simulink model "Assignment2_group37"  (R2023b)
settings: Solver=FixedStepAuto  StartTime=0.0  StopTime=10.0  FixedStep=1e-3  RelTol=1e-3  EnableMultiTasking=on
undefined symbols (not defined in the file): a, A0, A1, b, c, D0, D1, D10, D11, D12, D13, D2, D3, D4, D5, D6, D7, D8, D9, magnitude, PTA0, PTA1, PTA2, PTB2, PTB23, PTB3, PTB9, PTC16, PTC17, PTC2, PTC3, PTC4, PTD0, PTD1, PTD2, PTD3
libraries: frdmk64flib x19, etargetslib x2, dspstat3 x1, hdlsllib x1
settings Model: ExtModeTrigDuration=5  Creator=aless  LastModifiedBy=aless
settings OptimizationCC: EnhancedBackFolding=on  PassReuseOutputArgsAs=Individual arguments  ZeroExternalMemoryAtStartup=off  ZeroInternalMemoryAtStartup=off  MaxStackSize=64  OptimizeBlockOrder=speed  DifferentSizesBufferReuse=on  OptimizationCustomize=off  EfficientTunableParamExpr=on
settings DebuggingCC: ParameterTunabilityLossMsg=error
settings HardwareCC: ProdBitPerPointer=32  ProdBitPerSizeT=32  ProdBitPerPtrDiffT=32  ProdLargestAtomicInteger=Long  ProdLargestAtomicFloat=Double  ProdWordSize=32  ProdHWDeviceType=ARM Compatible->ARM Cortex
settings SFSimCC: MATLABDynamicMemAlloc=off
settings RTWCC: Description=Embedded Coder  SystemTargetFile=ert.tlc  HardwareBoard=NXP FRDM-K64F  TLCOptions="-aInlineSetEventsForThisBaseRateFcn=TLC_FALSE -aSuppressMultiTaskScheduler=TLC_FALSE  -aRateBasedStepFcn=0"  TemplateMakefile=ert_default_tmf  Toolchain=GNU Tools for ARM Embedded Processors
settings CodeAppCC: ForceParamTrailComments=on  IgnoreCustomStorageClasses=off  OperatorAnnotations=on  SimulinkDataObjDesc=on  SFDataObjDesc=on  InsertBlockDesc=on
settings ERTTargetCC: ExtModeTransport=4  ExtModeMexFile=sendToCommService

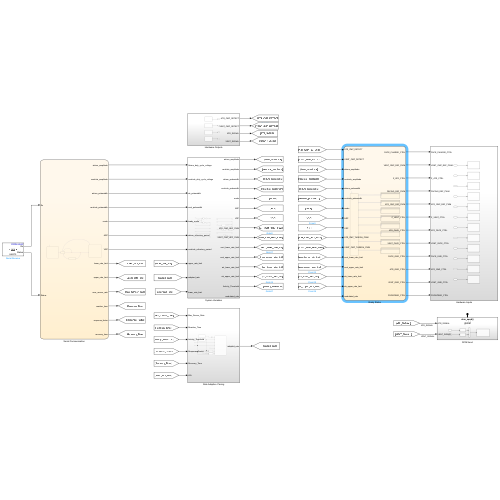
[thumbnail: Simulink's stored preview of the top-level diagram]
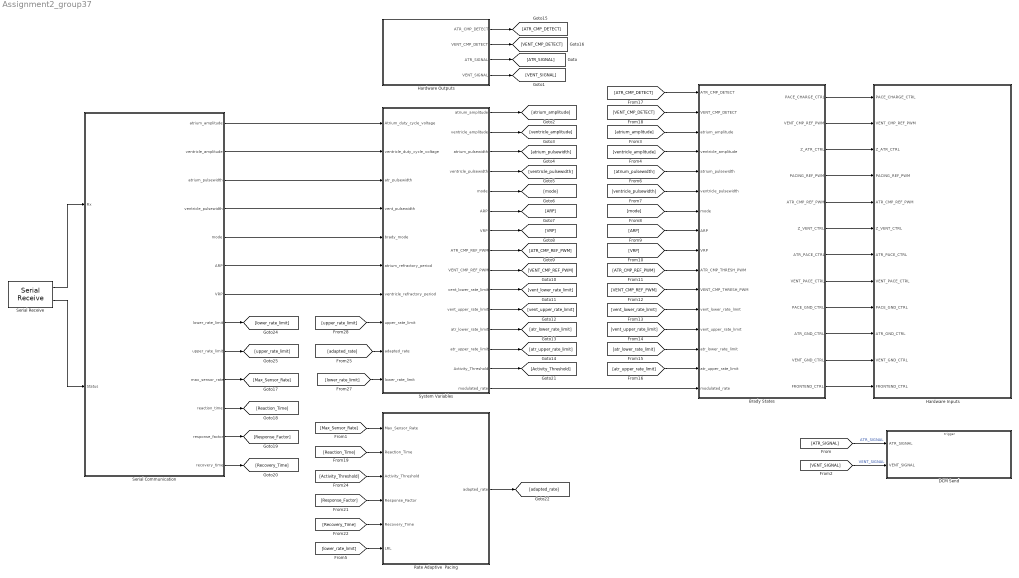
== system Assignment2_group37 ==
  Brady States : Stateflow chart  TreatAsAtomicUnit=on
      settings: PortSchema="{\"entries\":[{\"content\":{\"sides\":[{\"content\":{\"connectorIds\":[\"In1\",\"In2\",\"In3\",\"In4\",\"In5\",\"In6\",\"In7\",\"In8\",\"In9\",\"In10\",\"In11\",\"In12\",\"In13\",\"In14\",\"In15\",\"In16\"]},\"type\":\"ConnectorPlacement.EquallySpacedRectSide\",\"uuid\":\"d1839c8f-6221-46d4-ade1-365648b0880c\"},{\"content\":{\"connectorIds\":[\"Out1\",\"Out2\",\"Out3\",\"Out4\",\"Out5\",\"Out6\",\"Out7\",\"Out8\",\"Out9\",\"Out12\",\"Out10\",\"Out11\"],\"side\":\"RIGHT\"},\"type\":\"ConnectorPlacement.EquallySpacedRectSide\",\"uuid\":\"5469c751-f649-49a4-acaa-2051f4899f66\"},{\"content\":{\"side\":\"TOP\"},\"type\":\"ConnectorPlacement.EquallySpacedRectSide\",\"uuid\":\"ee663bab-8db3-49ac-8698-0304788d9d5e\"},{\"content\":{\"side\":\"BOTTOM\"},\"type\":\"ConnectorPlacement.EquallySpacedRectSide\",\"uuid\":\"7b3ff5b2-4ab8-41cc-b0f7-2e83bde3fafa\"}]},\"type\":\"ConnectorPlacement.EquallySpacedConnector\",\"uuid\":\"0582f962-be2e-4f7f-ab84-ab175671d8de\"}],\"packageUris\":[\"http://schema.mathworks.com/mf0/Connector/R2020b\"],\"version\":\"1.0\"}"
  DCM Send : Subsystem
  Hardware Inputs : Subsystem
  Hardware Outputs : Subsystem
  Rate Adaptive  Pacing : Subsystem
  Serial Communication : Stateflow chart  TreatAsAtomicUnit=on
  Serial Receive : frdmk64flib/Serial Receive  SCIModule=0  Baudrate=uint32(9600)  Parity=None  StopBits=1  HardwareFlowControl=None  ByteOrder=LittleEndian  DataType=uint8  DataLength=48  BlockingMode=off  OutputStatus=on  SampleTime=-1
  System Variables : Subsystem
  wires:
  Brady States/9(PACE_GND_CTRL) -> Hardware Inputs/9(PACE_GND_CTRL)
  Brady States/3(Z_ATR_CTRL) -> Hardware Inputs/3(Z_ATR_CTRL)
  Hardware Outputs/4(VENT_SIGNAL) -> [VENT_SIGNAL]
  Hardware Outputs/3(ATR_SIGNAL) -> [ATR_SIGNAL]
  [Recovery_Time] -> Rate Adaptive  Pacing/5(Recovery_Time)
  [adapted_rate] -> System Variables/9(adapted_rate)
  Serial Receive/1 -> Serial Communication/1(Rx)
  Serial Communication/2(ventricle_amplitude) -> System Variables/2(ventricle_duty_cycle_voltage)
  Serial Communication/7(VRP) -> System Variables/7(ventricle_refractory_period)
  System Variables/8(ATR_CMP_REF_PWM) -> [ATR_CMP_REF_PWM]
  System Variables/7(VRP) -> [VRP]
  System Variables/4(ventricle_pulsewidth) -> [ventricle_pulsewidth]
  System Variables/1(atrium_amplitude) -> [atrium_amplitude]
  [mode] -> Brady States/7(mode)
  System Variables/15(modulated_rate) -> Brady States/16(modulated_rate)
  System Variables/13(atr_upper_rate_limit) -> [atr_upper_rate_limit]
  System Variables/12(atr_lower_rate_limit) -> [atr_lower_rate_limit]
  Brady States/11(FRONTEND_CTRL) -> Hardware Inputs/12(FRONTEND_CTRL)
  Brady States/12(ATR_GND_CTRL) -> Hardware Inputs/10(ATR_GND_CTRL)
  Brady States/8(VENT_PACE_CTRL) -> Hardware Inputs/8(VENT_PACE_CTRL)
  Brady States/7(ATR_PACE_CTRL) -> Hardware Inputs/7(ATR_PACE_CTRL)
  Brady States/2(VENT_CMP_REF_PWM) -> Hardware Inputs/2(VENT_CMP_REF_PWM)
  [ventricle_pulsewidth] -> Brady States/6(ventricle_pulsewidth)
  [ventricle_amplitude] -> Brady States/4(ventricle_amplitude)
  [atr_upper_rate_limit] -> Brady States/15(atr_upper_rate_limit)
  [atr_lower_rate_limit] -> Brady States/14(atr_lower_rate_limit)
  Brady States/10(VENT_GND_CTRL) -> Hardware Inputs/11(VENT_GND_CTRL)
  System Variables/3(atrium_pulsewidth) -> [atrium_pulsewidth]
  System Variables/2(ventricle_amplitude) -> [ventricle_amplitude]
  [Reaction_Time] -> Rate Adaptive  Pacing/2(Reaction_Time)
  [upper_rate_limit] -> System Variables/8(upper_rate_limit)
  [ARP] -> Brady States/8(ARP)
  Hardware Outputs/1(ATR_CMP_DETECT) -> [ATR_CMP_DETECT]
  System Variables/9(VENT_CMP_REF_PWM) -> [VENT_CMP_REF_PWM]
  [Activity_Threshold] -> Rate Adaptive  Pacing/3(Activity_Threshold)
  Brady States/6(Z_VENT_CTRL) -> Hardware Inputs/6(Z_VENT_CTRL)
  Brady States/4(PACING_REF_PWM) -> Hardware Inputs/4(PACING_REF_PWM)
  Serial Communication/13(recovery_time) -> [Recovery_Time]
  System Variables/5(mode) -> [mode]
  [ATR_CMP_DETECT] -> Brady States/1(ATR_CMP_DETECT)
  Serial Communication/10(max_sensor_rate) -> [Max_Sensor_Rate]
  [atrium_pulsewidth] -> Brady States/5(atrium_pulsewidth)
  Serial Communication/3(atrium_pulsewidth) -> System Variables/3(atr_pulsewidth)
  [Max_Sensor_Rate] -> Rate Adaptive  Pacing/1(Max_Sensor_Rate)
  [VENT_CMP_DETECT] -> Brady States/2(VENT_CMP_DETECT)
  System Variables/6(ARP) -> [ARP]
  Brady States/5(ATR_CMP_REF_PWM) -> Hardware Inputs/5(ATR_CMP_REF_PWM)
  System Variables/11(vent_upper_rate_limit) -> [vent_upper_rate_limit]
  [VENT_CMP_REF_PWM] -> Brady States/11(VENT_CMP_THRESH_PWM)
  [lower_rate_limit] -> System Variables/10(lower_rate_limit)
  Serial Receive/2 -> Serial Communication/2(Status)
  Serial Communication/4(ventricle_pulsewidth) -> System Variables/4(vent_pulsewidth)
  System Variables/10(vent_lower_rate_limit) -> [vent_lower_rate_limit]
  [Response_Factor] -> Rate Adaptive  Pacing/4(Response_Factor)
  Rate Adaptive  Pacing/1(adapted_rate) -> [adapted_rate]
  Hardware Outputs/2(VENT_CMP_DETECT) -> [VENT_CMP_DETECT]
  [VRP] -> Brady States/9(VRP)
  Serial Communication/1(atrium_amplitude) -> System Variables/1(Atrium_duty_cycle_voltage)
  [lower_rate_limit] -> Rate Adaptive  Pacing/6(LRL)
  Serial Communication/12(response_factor) -> [Response_Factor]
  Serial Communication/11(reaction_time) -> [Reaction_Time]
  Serial Communication/8(lower_rate_limit) -> [lower_rate_limit]
  Serial Communication/5(mode) -> System Variables/5(brady_mode)
  [ATR_SIGNAL] -> DCM Send/1(ATR_SIGNAL)  "ATR_SIGNAL"
  Brady States/1(PACE_CHARGE_CTRL) -> Hardware Inputs/1(PACE_CHARGE_CTRL)
  [VENT_SIGNAL] -> DCM Send/2(VENT_SIGNAL)  "VENT_SIGNAL"
  [vent_upper_rate_limit] -> Brady States/13(vent_upper_rate_limit)
  [vent_lower_rate_limit] -> Brady States/12(vent_lower_rate_limit)
  [ATR_CMP_REF_PWM] -> Brady States/10(ATR_CMP_THRESH_PWM)
  [atrium_amplitude] -> Brady States/3(atrium_amplitude)
  System Variables/14(Activity_Threshold) -> [Activity_Threshold]
  Serial Communication/6(ARP) -> System Variables/6(atrium_refractory_period)
  Serial Communication/9(upper_rate_limit) -> [upper_rate_limit]

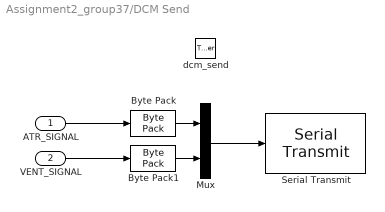
== system Assignment2_group37/DCM Send ==
  ATR_SIGNAL : Inport
  VENT_SIGNAL : Inport  Port=2
  dcm_send : TriggerPort  TriggerType=function-call  IsSimulinkFunction=on  FunctionName=dcm_send  VariantControl=Variant
  Byte Pack : etargetslib/Byte Pack  datatypes={'double'}  byteAlign=1
  Byte Pack1 : etargetslib/Byte Pack  datatypes={'double'}  byteAlign=1
  Mux : Mux  Inputs=2
  Serial Transmit : frdmk64flib/Serial Transmit  SCIModule=0  Baudrate=uint32(9600)  Parity=None  StopBits=1  HardwareFlowControl=None  ByteOrder=LittleEndian  BlockingMode=on  OutputStatus=on
  wires:
  Byte Pack/1 -> Mux/1
  Byte Pack1/1 -> Mux/2
  Mux/1 -> Serial Transmit/1
  ATR_SIGNAL/1 -> Byte Pack/1
  VENT_SIGNAL/1 -> Byte Pack1/1

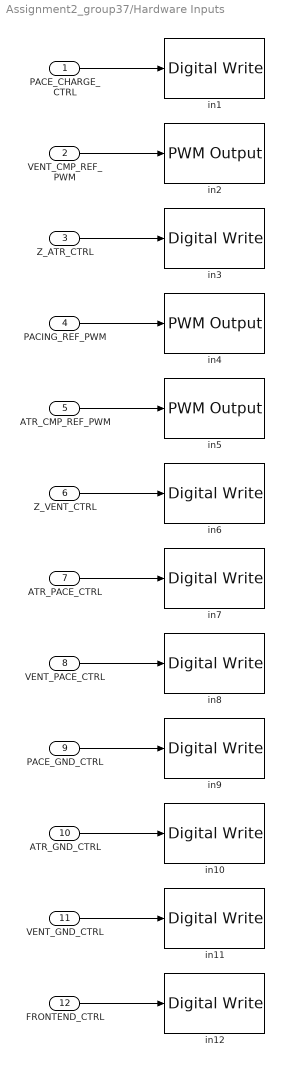
== system Assignment2_group37/Hardware Inputs ==
  PACE_CHARGE_CTRL : Inport
  VENT_CMP_REF_PWM : Inport  Port=2
  Z_ATR_CTRL : Inport  Port=3
  PACING_REF_PWM : Inport  Port=4
  ATR_CMP_REF_PWM : Inport  Port=5
  Z_VENT_CTRL : Inport  Port=6
  ATR_PACE_CTRL : Inport  Port=7
  VENT_PACE_CTRL : Inport  Port=8
  PACE_GND_CTRL : Inport  Port=9
  ATR_GND_CTRL : Inport  Port=10
  VENT_GND_CTRL : Inport  Port=11
  FRONTEND_CTRL : Inport  Port=12
  in1 : frdmk64flib/Digital Write  Whichpin=PTB9 (D2)
  in10 : frdmk64flib/Digital Write  Whichpin=PTD2 (D11)
  in11 : frdmk64flib/Digital Write  Whichpin=PTD3 (D12)
  in12 : frdmk64flib/Digital Write  Whichpin=PTD1 (D13)
  in2 : frdmk64flib/PWM Output  Whichpin=PTA1 (D3)  InitialFrequency=2000  InitialDutyCycle=30
  in3 : frdmk64flib/Digital Write  Whichpin=PTB23 (D4)
  in4 : frdmk64flib/PWM Output  Whichpin=PTA2 (D5)  InitialFrequency=2000  InitialDutyCycle=30
  in5 : frdmk64flib/PWM Output  Whichpin=PTC2 (D6)  InitialFrequency=2000  InitialDutyCycle=30
  in6 : frdmk64flib/Digital Write  Whichpin=PTC3 (D7)
  in7 : frdmk64flib/Digital Write  Whichpin=PTA0 (D8)
  in8 : frdmk64flib/Digital Write  Whichpin=PTC4 (D9)
  in9 : frdmk64flib/Digital Write  Whichpin=PTD0 (D10)
  wires:
  ATR_GND_CTRL/1 -> in10/1
  PACING_REF_PWM/1 -> in4/1
  Z_VENT_CTRL/1 -> in6/1
  VENT_GND_CTRL/1 -> in11/1
  VENT_PACE_CTRL/1 -> in8/1
  ATR_CMP_REF_PWM/1 -> in5/1
  FRONTEND_CTRL/1 -> in12/1
  PACE_CHARGE_CTRL/1 -> in1/1
  ATR_PACE_CTRL/1 -> in7/1
  PACE_GND_CTRL/1 -> in9/1
  Z_ATR_CTRL/1 -> in3/1
  VENT_CMP_REF_PWM/1 -> in2/1

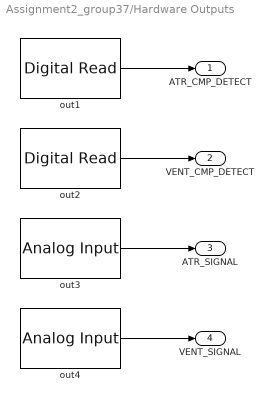
== system Assignment2_group37/Hardware Outputs ==
  out1 : frdmk64flib/Digital Read  Whichpin=PTC16 (D0)  SampleTime=-1
  out2 : frdmk64flib/Digital Read  Whichpin=PTC17 (D1)  SampleTime=-1
  out3 : frdmk64flib/Analog Input  Whichpin=PTB2 (A0)  SampleTime=-1
  out4 : frdmk64flib/Analog Input  Whichpin=PTB3 (A1)  SampleTime=-1
  ATR_CMP_DETECT : Outport
  VENT_CMP_DETECT : Outport  Port=2
  ATR_SIGNAL : Outport  Port=3
  VENT_SIGNAL : Outport  Port=4
  wires:
  out1/1 -> ATR_CMP_DETECT/1
  out2/1 -> VENT_CMP_DETECT/1
  out3/1 -> ATR_SIGNAL/1
  out4/1 -> VENT_SIGNAL/1

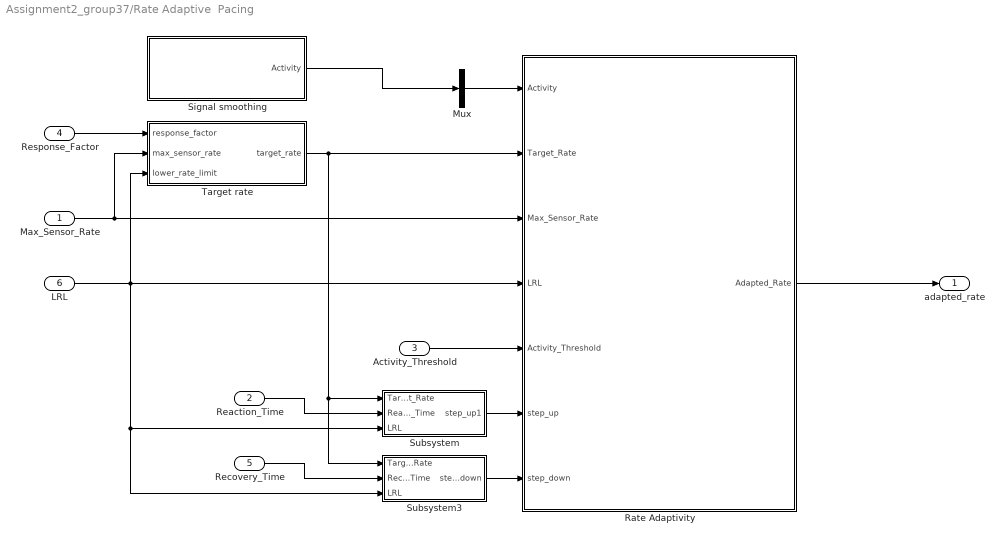
== system Assignment2_group37/Rate Adaptive  Pacing ==
  Max_Sensor_Rate : Inport
  Reaction_Time : Inport  Port=2
  Activity_Threshold : Inport  Port=3
  Response_Factor : Inport  Port=4
  Recovery_Time : Inport  Port=5
  LRL : Inport  Port=6
  Mux : Mux  Inputs=1
  Rate Adaptivity : Stateflow chart  TreatAsAtomicUnit=on
  Signal smoothing : Subsystem
  Subsystem : Subsystem
  Subsystem3 : Subsystem
  Target rate : Subsystem
  adapted_rate : Outport
  wires:
  Activity_Threshold/1 -> Rate Adaptivity/5(Activity_Threshold)
  Mux/1 -> Rate Adaptivity/1(Activity)
  Response_Factor/1 -> Target rate/1(response_factor)
  Signal smoothing/1(Activity) -> Mux/1
  Reaction_Time/1 -> Subsystem/2(Reaction_Time)
  Max_Sensor_Rate/1 -> Target rate/2(max_sensor_rate), Rate Adaptivity/3(Max_Sensor_Rate)
  LRL/1 -> Rate Adaptivity/4(LRL), Subsystem/3(LRL), Subsystem3/3(LRL), Target rate/3(lower_rate_limit)
  Subsystem/1(step_up1) -> Rate Adaptivity/6(step_up)
  Recovery_Time/1 -> Subsystem3/2(Recovery_Time)
  Subsystem3/1(step_down) -> Rate Adaptivity/7(step_down)
  Rate Adaptivity/1(Adapted_Rate) -> adapted_rate/1
  Target rate/1(target_rate) -> Rate Adaptivity/2(Target_Rate), Subsystem3/1(Target_Rate), Subsystem/1(Target_Rate)

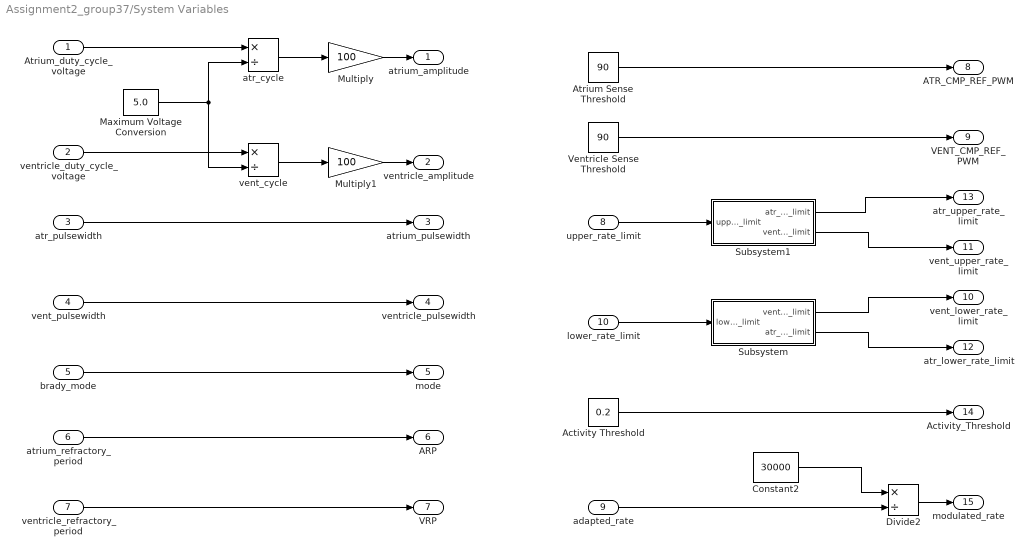
== system Assignment2_group37/System Variables ==
  Atrium_duty_cycle_voltage : Inport
  ventricle_duty_cycle_voltage : Inport  Port=2
  atr_pulsewidth : Inport  Port=3
  vent_pulsewidth : Inport  Port=4
  brady_mode : Inport  Port=5  PortDimensions=8
  atrium_refractory_period : Inport  Port=6
  ventricle_refractory_period : Inport  Port=7
  upper_rate_limit : Inport  Port=8
  adapted_rate : Inport  Port=9
  lower_rate_limit : Inport  Port=10  OutDataTypeStr=double
  Activity Threshold : Constant  Value=0.2  OutDataTypeStr=double
  Atrium Sense Threshold : Constant  Value=90
  Constant2 : Constant  Value=30000
  Divide2 : Product  Inputs=*/
  Maximum Voltage Conversion : Constant  Value=5.0
  Multiply : Gain  Gain=100
  Multiply1 : Gain  Gain=100
  Subsystem : Subsystem
  Subsystem1 : Subsystem
  Ventricle Sense Threshold : Constant  Value=90
  atr_cycle : Product  Inputs=*/
  vent_cycle : Product  Inputs=*/
  atrium_amplitude : Outport
  ventricle_amplitude : Outport  Port=2
  atrium_pulsewidth : Outport  Port=3  OutDataTypeStr=double
  ventricle_pulsewidth : Outport  Port=4  OutDataTypeStr=double
  mode : Outport  Port=5  PortDimensions=8
  ARP : Outport  Port=6  OutDataTypeStr=double
  VRP : Outport  Port=7  OutDataTypeStr=double
  ATR_CMP_REF_PWM : Outport  Port=8
  VENT_CMP_REF_PWM : Outport  Port=9
  vent_lower_rate_limit : Outport  Port=10
  vent_upper_rate_limit : Outport  Port=11
  atr_lower_rate_limit : Outport  Port=12
  atr_upper_rate_limit : Outport  Port=13
  Activity_Threshold : Outport  Port=14
  modulated_rate : Outport  Port=15
  wires:
  atr_cycle/1 -> Multiply/1
  vent_cycle/1 -> Multiply1/1
  Maximum Voltage Conversion/1 -> vent_cycle/2, atr_cycle/2
  brady_mode/1 -> mode/1
  Atrium_duty_cycle_voltage/1 -> atr_cycle/1
  ventricle_duty_cycle_voltage/1 -> vent_cycle/1
  Atrium Sense Threshold/1 -> ATR_CMP_REF_PWM/1
  Ventricle Sense Threshold/1 -> VENT_CMP_REF_PWM/1
  Activity Threshold/1 -> Activity_Threshold/1
  Multiply1/1 -> ventricle_amplitude/1
  Multiply/1 -> atrium_amplitude/1
  lower_rate_limit/1 -> Subsystem/1(lower_rate_limit)
  Subsystem/1(vent_lower_rate_limit) -> vent_lower_rate_limit/1
  ventricle_refractory_period/1 -> VRP/1
  atrium_refractory_period/1 -> ARP/1
  atr_pulsewidth/1 -> atrium_pulsewidth/1
  vent_pulsewidth/1 -> ventricle_pulsewidth/1
  Subsystem/2(atr_lower_rate_limit) -> atr_lower_rate_limit/1
  adapted_rate/1 -> Divide2/2
  Constant2/1 -> Divide2/1
  Divide2/1 -> modulated_rate/1
  upper_rate_limit/1 -> Subsystem1/1(upper_rate_limit)
  Subsystem1/1(atr_upper_rate_limit) -> atr_upper_rate_limit/1
  Subsystem1/2(vent_upper_rate_limit) -> vent_upper_rate_limit/1

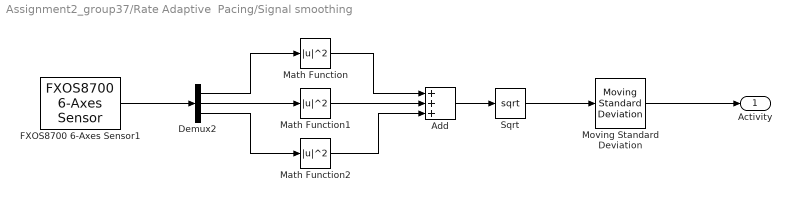
== system Assignment2_group37/Rate Adaptive  Pacing/Signal smoothing ==
  Add : Sum  Inputs=+++
  Demux2 : Demux  Outputs=3
  FXOS8700 6-Axes Sensor1 : frdmk64flib/FXOS8700 6-Axes Sensor  Activesensor=Accelerometer only  ODR=100Hz  HybridODR=400Hz  Accelfullrange=-4g to +4g  SampleTime=1/100
  Math Function : Math  Operator=magnitude^2  SignedPower=on  OutDataTypeStr=double
  Math Function1 : Math  Operator=magnitude^2  SignedPower=on  OutDataTypeStr=double
  Math Function2 : Math  Operator=magnitude^2  SignedPower=on  OutDataTypeStr=double
  Moving Standard Deviation : dspstat3/Moving Standard Deviation  Method=Sliding window  ForgettingFactorPort=off  SpecifyWindowLength=on  WindowLength=128  OverlapLength=127  AllowArbitraryInputLength=off  ForgettingFactor=0.9  SimulateUsing=Code generation
  Sqrt : Sqrt
  Activity : Outport  SourceOfInitialOutputValue=Input signal
  wires:
  Sqrt/1 -> Moving Standard Deviation/1
  FXOS8700 6-Axes Sensor1/1 -> Demux2/1
  Math Function/1 -> Add/1
  Add/1 -> Sqrt/1
  Math Function2/1 -> Add/3
  Demux2/2 -> Math Function1/1
  Math Function1/1 -> Add/2
  Demux2/1 -> Math Function/1
  Demux2/3 -> Math Function2/1
  Moving Standard Deviation/1 -> Activity/1

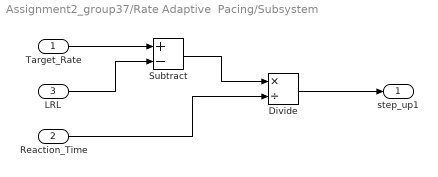
== system Assignment2_group37/Rate Adaptive  Pacing/Subsystem ==
  Target_Rate : Inport
  Reaction_Time : Inport  Port=2
  LRL : Inport  Port=3
  Divide : Product  Inputs=*/
  Subtract : Sum  Inputs=+-
  step_up1 : Outport
  wires:
  Subtract/1 -> Divide/1
  Divide/1 -> step_up1/1
  Target_Rate/1 -> Subtract/1
  LRL/1 -> Subtract/2
  Reaction_Time/1 -> Divide/2

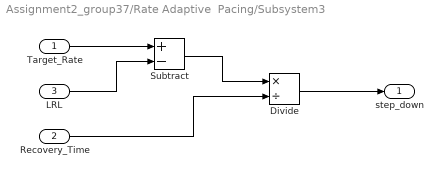
== system Assignment2_group37/Rate Adaptive  Pacing/Subsystem3 ==
  Target_Rate : Inport
  Recovery_Time : Inport  Port=2
  LRL : Inport  Port=3
  Divide : Product  Inputs=*/
  Subtract : Sum  Inputs=+-
  step_down : Outport
  wires:
  Subtract/1 -> Divide/1
  Divide/1 -> step_down/1
  Target_Rate/1 -> Subtract/1
  LRL/1 -> Subtract/2
  Recovery_Time/1 -> Divide/2

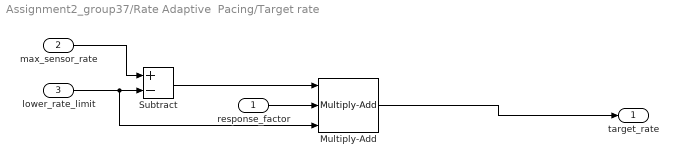
== system Assignment2_group37/Rate Adaptive  Pacing/Target rate ==
  response_factor : Inport
  max_sensor_rate : Inport  Port=2
  lower_rate_limit : Inport  Port=3
  Multiply-Add : hdlsllib/HDL Operations/Multiply-Add  Function=c+(a.*b)  datatype=uint16  RndMeth=Nearest  DoSatur=off  FMA=off
  Subtract : Sum  Inputs=+-
  target_rate : Outport  OutDataTypeStr=uint16  SourceOfInitialOutputValue=Input signal
  wires:
  max_sensor_rate/1 -> Subtract/1
  lower_rate_limit/1 -> Multiply-Add/3, Subtract/2
  Subtract/1 -> Multiply-Add/1
  response_factor/1 -> Multiply-Add/2
  Multiply-Add/1 -> target_rate/1

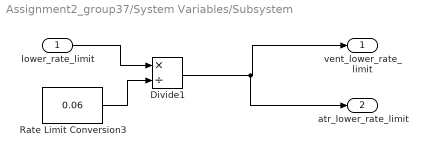
== system Assignment2_group37/System Variables/Subsystem ==
  lower_rate_limit : Inport
  Divide1 : Product  Inputs=*/
  Rate Limit Conversion3 : Constant  Value=0.06
  vent_lower_rate_limit : Outport
  atr_lower_rate_limit : Outport  Port=2
  wires:
  Divide1/1 -> atr_lower_rate_limit/1, vent_lower_rate_limit/1
  lower_rate_limit/1 -> Divide1/1
  Rate Limit Conversion3/1 -> Divide1/2

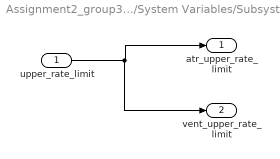
== system Assignment2_group37/System Variables/Subsystem1 ==
  upper_rate_limit : Inport
  atr_upper_rate_limit : Outport
  vent_upper_rate_limit : Outport  Port=2
  wires:
  upper_rate_limit/1 -> vent_upper_rate_limit/1, atr_upper_rate_limit/1

== stateflow chart Assignment2_group37/Serial Communication ==
  state SET_PARAM
    entry:
    mode = typecast(Rx(3:4), 'uint16');
    lower_rate_limit = typecast(Rx(5:6), 'uint16');
    upper_rate_limit = typecast(Rx(7:8), 'uint16');
    ventricle_amplitude = typecast(Rx(9:16), 'double');
    ventricle_pulsewidth = typecast(Rx(17:18), 'uint16');
    VRP = typecast(Rx(19:20), 'uint16');
    atrium_amplitude = typecast(Rx(21:28), 'double');
    atrium_pulsewidth = typecast(Rx(29:30), 'uint16');
    ARP = typecast(Rx(39:40), 'uint16');
    max_sensor_rate = typecast(Rx(41:42), 'uint16');
    reaction_time = typecast(Rx(43:44), 'uint16');
    response_factor = typecast(Rx(45:46), 'uint16');;
    recovery_time = typecast(Rx(47:48), 'uint16');
    update = 1;
  state Initial
    entry:
    mode = 0;
    lower_rate_limit = 60;
    upper_rate_limit = 120;
    reaction_time = 10;
    response_factor = 16;
    recovery_time = 20;
    max_sensor_rate = 180;
    atrium_amplitude = 3.5;
    atrium_pulsewidth = 10;
    ARP = 200;
    ventricle_amplitude = 3.5;
    ventricle_pulsewidth = 10;
    VRP = 200;
  state STANDBY
  state TRANSITION
    entry:
    dcm_send();
  SET_PARAM -> STANDBY
  (default) -> Initial
  (junction 82) -> STANDBY [order 2]
  Initial -> STANDBY
  STANDBY -> (junction 82) : [Status == 0]
  (junction 82) -> (junction 68) [order 1] : [Rx(1) == hex2dec('16')]
  (junction 68) -> SET_PARAM [order 2] : [Rx(2) == hex2dec('55')]
  (junction 68) -> TRANSITION [order 1] : [Rx(2) == hex2dec('22')]
  TRANSITION -> STANDBY
  data: Rx input uint8; Status input uint8; atrium_amplitude output single size=8; ventricle_amplitude output single; atrium_pulsewidth output single; ventricle_pulsewidth output single; mode output uint16; ARP output uint16; VRP output uint16; lower_rate_limit output uint16; upper_rate_limit output uint16; max_sensor_rate output uint16; reaction_time output uint16; response_factor output uint16; recovery_time output uint16

== stateflow chart Assignment2_group37/Brady States ==
  state AOO [group]
    state Charging
      entry:
      %Charge C22
      ATR_PACE_CTRL = false
      VENT_PACE_CTRL = false
      PACING_REF_PWM = atrium_amplitude
      PACE_CHARGE_CTRL = true
      %Discharge C21
      PACE_GND_CTRL = true
      VENT_PACE_CTRL = false
      Z_ATR_CTRL = false
      Z_VENT_CTRL = false
      ATR_PACE_CTRL = false
      ATR_GND_CTRL = true
      VENT_GND_CTRL = false
    state Discharging
      entry:
      %Discharge C22 to charge C21
      PACE_CHARGE_CTRL = false
      PACE_GND_CTRL = true
      VENT_PACE_CTRL = false
      VENT_GND_CTRL = false
      Z_VENT_CTRL = false
      Z_ATR_CTRL = false
      ATR_GND_CTRL = false
      ATR_PACE_CTRL = true
    AOO.Charging -> AOO.Discharging [order 1] : after((60000/atrium_lower_rate_limit)- atrium_pulsewidth,msec)
    AOO.Discharging -> AOO.Charging : after((atrium_pulsewidth),msec)
  state Mode
  state VOO [group]
    state Discharging
      entry:
      %discharge C22 to charge C21
      PACE_CHARGE_CTRL = false
      PACE_GND_CTRL = true
      ATR_PACE_CTRL = false
      ATR_GND_CTRL = false
      Z_VENT_CTRL = false
      Z_ATR_CTRL = false
      VENT_GND_CTRL = false
      VENT_PACE_CTRL = true
    state Charging
      entry:
      %charge C22
      ATR_PACE_CTRL = false
      VENT_PACE_CTRL = false
      PACING_REF_PWM = ventricle_amplitude
      PACE_CHARGE_CTRL = true
      %discharge C21 into ventricle ground
      PACE_GND_CTRL = true
      VENT_PACE_CTRL = false
      Z_ATR_CTRL = false
      Z_VENT_CTRL = false
      ATR_PACE_CTRL = false
      ATR_GND_CTRL = false
      VENT_GND_CTRL = true
    note: after((ventricle_pulsewidth),msec)
    VOO.Discharging -> VOO.Charging
    VOO.Charging -> VOO.Discharging [order 1] : after((60000/ventricle_lower_rate_limit)-ventricle_pulsewidth,msec)
  state AAI [group]
    state Charging
      entry:
      %Turn on sensing
      FRONTEND_CTRL = true
      ATR_CMP_REF_PWM = ATR_CMP_THRESH_PWM
      %Charging capacitor C22
      ATR_PACE_CTRL = false
      VENT_PACE_CTRL = false
      PACING_REF_PWM = atrium_amplitude
      PACE_CHARGE_CTRL = true
      %Discharge C21 into Atrium ground
      PACE_GND_CTRL = true
      VENT_PACE_CTRL = false
      Z_ATR_CTRL = false
      Z_VENT_CTRL = false
      ATR_PACE_CTRL = false
      ATR_GND_CTRL = true
      VENT_GND_CTRL = false
    state Discharging
      entry:
      %discharge C22 to charge C21
      PACE_CHARGE_CTRL = false
      PACE_GND_CTRL = true
      VENT_PACE_CTRL = false
      VENT_GND_CTRL = false
      Z_VENT_CTRL = false
      Z_ATR_CTRL = false
      ATR_GND_CTRL = false
      ATR_PACE_CTRL = true
    state Transition
      %Check for sense outside atrium refractory period
    AAI.Discharging -> AAI.Charging : after(atrium_pulsewidth, msec)
    AAI.Charging -> AAI.Transition [order 1] : after(ARP, msec)
    AAI.Transition -> AAI.Discharging [order 2] : after((60000/atrium_lower_rate_limit) - atrium_pulsewidth - ARP,msec)
    AAI.Transition -> AAI.Charging [order 1] : [ATR_CMP_DETECT == true]
  state VVI [group]
    state Charging
      entry:
      %Turn sensing on
      FRONTEND_CTRL = true
      VENT_CMP_REF_PWM = VENT_CMP_THRESH_PWM
      %Charging C22
      ATR_PACE_CTRL = false
      VENT_PACE_CTRL = false
      PACING_REF_PWM = ventricle_amplitude
      PACE_CHARGE_CTRL = true
      %Charge release of capacitor C21 into Ventricle ground
      PACE_GND_CTRL = true
      VENT_PACE_CTRL = false
      Z_ATR_CTRL = false
      Z_VENT_CTRL = false
      ATR_PACE_CTRL = false
      ATR_GND_CTRL = false
      VENT_GND_CTRL = true
    state Discharging
      entry:
      %discharge C22 to charge C21
      PACE_CHARGE_CTRL = false
      PACE_GND_CTRL = true
      ATR_PACE_CTRL = false
      ATR_GND_CTRL = false
      Z_VENT_CTRL = false
      Z_ATR_CTRL = false
      VENT_GND_CTRL = false
      VENT_PACE_CTRL = true
    state Transition
      %Check for sense outside atrium refractory period
    VVI.Discharging -> VVI.Charging : after(ventricle_pulsewidth, msec)
    VVI.Charging -> VVI.Transition [order 1] : after(VRP, msec)
    VVI.Transition -> VVI.Discharging [order 2] : after((60000/ventricle_lower_rate_limit) - ventricle_pulsewidth - VRP,msec)
    VVI.Transition -> VVI.Charging [order 1] : [VENT_CMP_DETECT == true]
  state AOOR [group]
    state Charging
      entry:
      %Charge C22
      ATR_PACE_CTRL = false
      VENT_PACE_CTRL = false
      PACING_REF_PWM = atrium_amplitude
      PACE_CHARGE_CTRL = true
      %Discharge C21
      PACE_GND_CTRL = true
      VENT_PACE_CTRL = false
      Z_ATR_CTRL = false
      Z_VENT_CTRL = false
      ATR_PACE_CTRL = false
      ATR_GND_CTRL = true
      VENT_GND_CTRL = false
    state Discharging
      entry:
      %Discharge C22 to charge C21
      PACE_CHARGE_CTRL = false
      PACE_GND_CTRL = true
      VENT_PACE_CTRL = false
      VENT_GND_CTRL = false
      Z_VENT_CTRL = false
      Z_ATR_CTRL = false
      ATR_GND_CTRL = false
      ATR_PACE_CTRL = true
    AOOR.Charging -> AOOR.Discharging [order 1] : after(modulated_rate - atrium_pulsewidth,msec)
    AOOR.Discharging -> AOOR.Charging : after((atrium_pulsewidth),msec)
  state VOOR [group]
    state Discharging
      entry:
      %discharge C22 to charge C21
      PACE_CHARGE_CTRL = false
      PACE_GND_CTRL = true
      ATR_PACE_CTRL = false
      ATR_GND_CTRL = false
      Z_VENT_CTRL = false
      Z_ATR_CTRL = false
      VENT_GND_CTRL = false
      VENT_PACE_CTRL = true
    state Charging
      entry:
      %charge C22
      ATR_PACE_CTRL = false
      VENT_PACE_CTRL = false
      PACING_REF_PWM = ventricle_amplitude
      PACE_CHARGE_CTRL = true
      %discharge C21 into ventricle ground
      PACE_GND_CTRL = true
      VENT_PACE_CTRL = false
      Z_ATR_CTRL = false
      Z_VENT_CTRL = false
      ATR_PACE_CTRL = false
      ATR_GND_CTRL = false
      VENT_GND_CTRL = true
    VOOR.Discharging -> VOOR.Charging : [after((ventricle_pulsewidth),msec)]
    VOOR.Charging -> VOOR.Discharging [order 1] : after((modulated_rate - ventricle_pulsewidth),msec)
  state AAIR [group]
    state Charging
      entry:
      %Turn on sensing
      FRONTEND_CTRL = true
      ATR_CMP_REF_PWM = ATR_CMP_THRESH_PWM
      %Charging capacitor C22
      ATR_PACE_CTRL = false
      VENT_PACE_CTRL = false
      PACING_REF_PWM = atrium_amplitude
      PACE_CHARGE_CTRL = true
      %Discharge C21 into Atrium ground
      PACE_GND_CTRL = true
      VENT_PACE_CTRL = false
      Z_ATR_CTRL = false
      Z_VENT_CTRL = false
      ATR_PACE_CTRL = false
      ATR_GND_CTRL = true
      VENT_GND_CTRL = false
    state Discharging
      entry:
      %discharge C22 to charge C21
      PACE_CHARGE_CTRL = false
      PACE_GND_CTRL = true
      VENT_PACE_CTRL = false
      VENT_GND_CTRL = false
      Z_VENT_CTRL = false
      Z_ATR_CTRL = false
      ATR_GND_CTRL = false
      ATR_PACE_CTRL = true
    state Transition
      %Check for sense outside atrium refractory period
    AAIR.Discharging -> AAIR.Charging : after(atrium_pulsewidth, msec)
    AAIR.Charging -> AAIR.Transition [order 1] : after(ARP, msec)
    AAIR.Transition -> AAIR.Discharging [order 2] : after((modulated_rate - atrium_pulsewidth - ARP ),msec)
    AAIR.Transition -> AAIR.Charging [order 1] : [ATR_CMP_DETECT == true]
  state VVIR [group]
    state Charging
      entry:
      %Turn sensing on
      FRONTEND_CTRL = true
      VENT_CMP_REF_PWM = VENT_CMP_THRESH_PWM
      %Charging C22
      ATR_PACE_CTRL = false
      VENT_PACE_CTRL = false
      PACING_REF_PWM = ventricle_amplitude
      PACE_CHARGE_CTRL = true
      %Charge release of capacitor C21 into Ventricle ground
      PACE_GND_CTRL = true
      VENT_PACE_CTRL = false
      Z_ATR_CTRL = false
      Z_VENT_CTRL = false
      ATR_PACE_CTRL = false
      ATR_GND_CTRL = false
      VENT_GND_CTRL = true
    state Discharging
      entry:
      %discharge C22 to charge C21
      PACE_CHARGE_CTRL = false
      PACE_GND_CTRL = true
      ATR_PACE_CTRL = false
      ATR_GND_CTRL = false
      Z_VENT_CTRL = false
      Z_ATR_CTRL = false
      VENT_GND_CTRL = false
      VENT_PACE_CTRL = true
    state Transition
      %Check for sense outside atrium refractory period
    VVIR.Discharging -> VVIR.Charging : after(ventricle_pulsewidth, msec)
    VVIR.Charging -> VVIR.Transition [order 1] : after(VRP, msec)
    VVIR.Transition -> VVIR.Discharging [order 2] : after((modulated_rate - ventricle_pulsewidth - VRP),msec)
    VVIR.Transition -> VVIR.Charging [order 1] : [VENT_CMP_DETECT == true]
  VOO.Charging -> Mode [order 2] : [mode~=1]
  AAI.Charging -> Mode [order 2] : [mode~=2]
  VVI.Charging -> Mode [order 2] : [mode~=3]
  VOOR.Charging -> Mode [order 2] : [mode~=5]
  AOOR.Charging -> Mode [order 2] : [mode~=4]
  AOO.Charging -> Mode [order 2] : [mode~=0]
  VVIR.Charging -> Mode [order 2] : [mode~=7]
  AAIR.Charging -> Mode [order 2] : [mode~=6]
  Mode -> AOOR.Charging [order 5] : [mode==4]
  Mode -> VOOR.Charging [order 6] : [mode==5]
  Mode -> AAIR.Charging [order 7] : [mode==6]
  Mode -> VVIR.Charging [order 8] : [mode==7]
  Mode -> VVI.Charging [order 4] : [mode==3]
  Mode -> AAI.Charging [order 3] : [mode==2]
  Mode -> VOO.Charging [order 2] : [mode==1]
  Mode -> AOO.Charging [order 1] : [mode==0]
  (default) -> Mode
  data: ATR_CMP_DETECT input; VENT_CMP_DETECT input; atrium_amplitude input; ventricle_amplitude input; atrium_pulsewidth input; ventricle_pulsewidth input; mode input; ARP input double; VRP input double; ATR_CMP_THRESH_PWM input; VENT_CMP_THRESH_PWM input; PACE_CHARGE_CTRL output; VENT_CMP_REF_PWM output; Z_ATR_CTRL output; PACING_REF_PWM output; ATR_CMP_REF_PWM output; Z_VENT_CTRL output; ATR_PACE_CTRL output; VENT_PACE_CTRL output; PACE_GND_CTRL output; VENT_GND_CTRL output; FRONTEND_CTRL output; ATR_GND_CTRL output; vent_lower_rate_limit input double; vent_upper_rate_limit input double; atr_lower_rate_limit input double; atr_upper_rate_limit input; modulated_rate input double

== stateflow chart Assignment2_group37/Rate Adaptive  Pacing/Rate Adaptivity ==
  state wait
  state Step_up
    entry:
    Adapted_Rate = stepu(Adapted_Rate, step_up);
  state Assign
    entry:
    Adapted_Rate = Target_Rate;
  state Start1
    entry:
    Adapted_Rate = LRL;
  state Step_down
    entry:
    Adapted_Rate = stepd(Adapted_Rate, step_up);
  state step_down2
    entry:
    Adapted_Rate = stepd(Adapted_Rate, step_down);
  state wait2
  wait -> Step_up : [after(1000,msec)]
  Step_up -> wait [order 1] : [[Adapted_Rate <= Target_Rate]]
  Step_up -> Assign [order 3] : [Adapted_Rate >= Target_Rate]
  Start1 -> Step_up [order 1] : [Activity >= Activity_Threshold]
  Step_up -> Step_down [order 2] : [Activity <  Activity_Threshold]
  Step_down -> Step_up [order 1] : [Activity >= Activity_Threshold]
  step_down2 -> Step_up [order 2] : [Activity >= Activity_Threshold]
  Assign -> Assign [order 2] : [Activity > Activity_Threshold]
  (default) -> Start1
  Assign -> step_down2 [order 1] : [Activity < Activity_Threshold]
  Step_down -> step_down2 [order 2] : [ after(1000,msec)]
  Start1 -> Start1 [order 2] : [Activity < Activity_Threshold]
  step_down2 -> Start1 [order 1] : [Adapted_Rate <= LRL]
  step_down2 -> wait2 [order 3] : [after(1000, msec)]
  wait2 -> step_down2 : [Adapted_Rate >= LRL]
  data: a function_input; b function_input; x function_output; a function_input; b function_input; x function_output; Activity input; Target_Rate input double; Max_Sensor_Rate input double; LRL input double; Activity_Threshold input double; Adapted_Rate output double; step_up input; step_down input; data local; data1 local
  function x = stepd(a,b):
    | function x = stepd(a,b)
    | x = a - b;
    | end
  function x = stepu(a,b):
    | function x = stepu(a,b)
    | x = a + b;
    | end
